simulink model "VLC_MULT"  (R2020a)
settings: Solver=VariableStepAuto  StartTime=0.0  StopTime=400  RelTol=1e-3
model workspace (MAT data in the model file):
  Name = 1
settings Model: Creator=JohnCarlo.Laude001  LastModifiedBy=JohnCarlo.Laude001

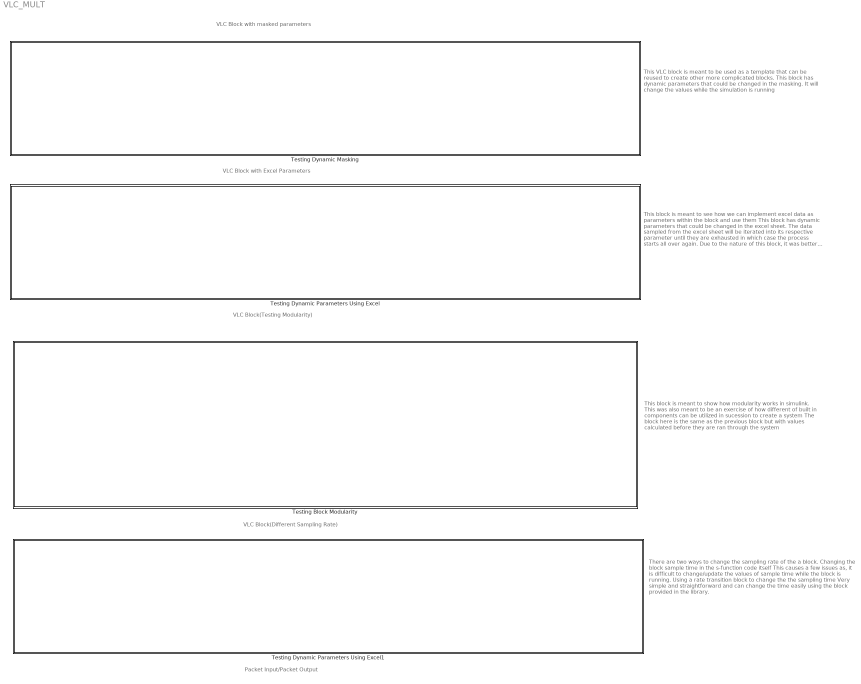
== system VLC_MULT ==
  note: This VLC block is meant to be used as a template that can be
      | reused to create other more complicated blocks.
      |
      | This block has dynamic parameters that could be changed in
      | the masking. It will change the values while the simulation is
      | running
  note: VLC Block with masked parameters
  note: VLC Block with Excel Parameters
  note: VLC Block(Testing Modularity)
  note: This block is meant to see how we can implement excel
      | data as parameters within the block and use them
      |
      | This block has dynamic parameters that could be changed in
      | the excel sheet. The data sampled from the excel sheet will be
      | iterated into its respective parameter until they are exhausted
      | in which case the process starts all over again. Due to the
      | nature of this block, it was better to run run the parameters
      | straight as inputs for ease of access instead of parameters.
  note: This block is meant to show how modularity works in simulink.
      | This was also meant to be an exercise of how different
      | of built in components can be utilized in sucession to
      | create a system
      |
      | The block here is the same as the previous block but with
      | values calculated before they are ran through the system
  note: VLC Block(Different Sampling Rate)
  note: There are two ways to change the sampling rate of the a block.
      | Changing the block sample time in the s-function code itself
      | This causes a few issues as, it is difficult to change/update
      | the values of sample time while the block is running.
      | Using a rate transition block to change the the sampling time
      | Very simple and straightforward and can change the time
      | easily using the block provided in the library.
  note: Packet Input/Packet Output
  Testing Block Modularity : Subsystem
  Testing Dynamic Masking : Subsystem
  Testing Dynamic Parameters Using Excel : Subsystem
  Testing Dynamic Parameters Using Excel1 : Subsystem

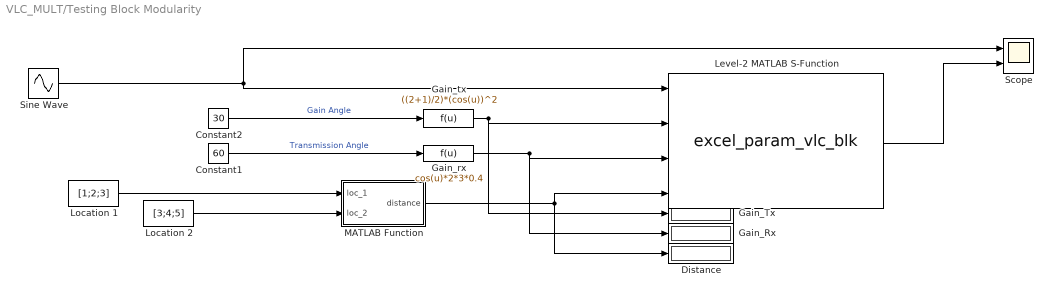
== system VLC_MULT/Testing Block Modularity ==
  Constant1 : Constant  Value=60
  Constant2 : Constant  Value=30
  Distance : Display
  Gain_Rx : Display
  Gain_Tx : Display
  Gain_rx : Fcn  Expr=cos(u)*2*3*0.4
  Gain_tx : Fcn  Expr=((2+1)/2)*(cos(u))^2
  Level-2 MATLAB S-Function : M-S-Function  FunctionName=excel_param_vlc_blk  Parameters=grx, gtx, d  mask{grx=90.0, gtx=100.0, d=100.0}
      mask prompts: grx "Gain Received"; gtx "Gain Transmission"; d "Distance"
      mask DialogControl DescGroupVar Prompt: VLC Block
      mask DialogControl DescTextVar Prompt: This block is meant to simulate the VLC system using the equation        H = (gain_tx*gain_rx)/(distance^2)
  Location 1 : Constant  Value=[1;2;3]
  Location 2 : Constant  Value=[3;4;5]
  MATLAB Function : MATLAB Function  TreatAsAtomicUnit=on
  Scope : Scope  NumInputPorts=2
  Sine Wave : Sin  SampleTime=0.001
  wires:
  Level-2 MATLAB S-Function/1 -> Scope/2
  Sine Wave/1 -> Scope/1, Level-2 MATLAB S-Function/1
  Gain_tx/1 -> Gain_Tx/1, Level-2 MATLAB S-Function/2
  Constant2/1 -> Gain_tx/1  "Gain Angle"
  Constant1/1 -> Gain_rx/1  "Transmission Angle"
  Gain_rx/1 -> Level-2 MATLAB S-Function/3, Gain_Rx/1
  Location 1/1 -> MATLAB Function/1(loc_1)
  MATLAB Function/1(distance) -> Level-2 MATLAB S-Function/4, Distance/1
  Location 2/1 -> MATLAB Function/2(loc_2)

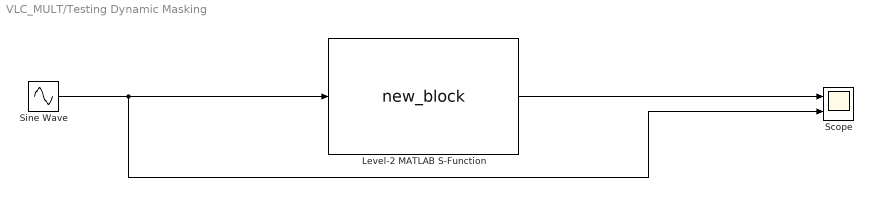
== system VLC_MULT/Testing Dynamic Masking ==
  Level-2 MATLAB S-Function : M-S-Function  FunctionName=new_block  Parameters=grx, gtx, d  mask{grx=81.0, gtx=41.0, d=78.0}
      mask prompts: grx "Gain Received"; gtx "Gain Transmission"; d "Distance"
      mask DialogControl DescGroupVar Prompt: VLC Block
      mask DialogControl DescTextVar Prompt: This block is meant to simulate the VLC system using the equation        H = (gain_tx*gain_rx)/(distance^2)
  Scope : Scope  NumInputPorts=2
  Sine Wave : Sin  SampleTime=0.001
  wires:
  Level-2 MATLAB S-Function/1 -> Scope/1
  Sine Wave/1 -> Scope/2, Level-2 MATLAB S-Function/1

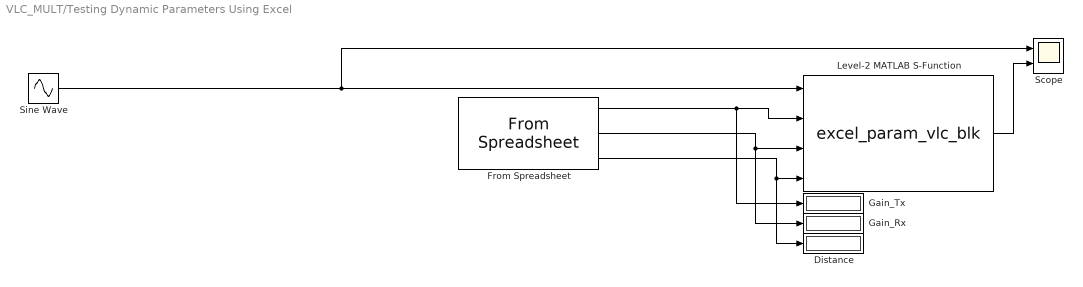
== system VLC_MULT/Testing Dynamic Parameters Using Excel ==
  Distance : Display
  From Spreadsheet : FromSpreadsheet  FileName=C:\Users\JohnCarlo.Laude001\Desktop\VLC_Research\VLC_Data_Test.xlsx  TreatFirstColumnAs=Data  SampleTime=50
  Gain_Rx : Display
  Gain_Tx : Display
  Level-2 MATLAB S-Function : M-S-Function  FunctionName=excel_param_vlc_blk  Parameters=grx, gtx, d  mask{grx=18.900, gtx=100.0, d=100.0}
      mask prompts: grx "Gain Received"; gtx "Gain Transmission"; d "Distance"
      mask DialogControl DescGroupVar Prompt: VLC Block
      mask DialogControl DescTextVar Prompt: This block is meant to simulate the VLC system using the equation        H = (gain_tx*gain_rx)/(distance^2)
  Scope : Scope  NumInputPorts=2
  Sine Wave : Sin  SampleTime=0.001
  wires:
  Sine Wave/1 -> Scope/1, Level-2 MATLAB S-Function/1
  From Spreadsheet/1 -> Gain_Tx/1, Level-2 MATLAB S-Function/2
  From Spreadsheet/2 -> Gain_Rx/1, Level-2 MATLAB S-Function/3
  From Spreadsheet/3 -> Distance/1, Level-2 MATLAB S-Function/4
  Level-2 MATLAB S-Function/1 -> Scope/2

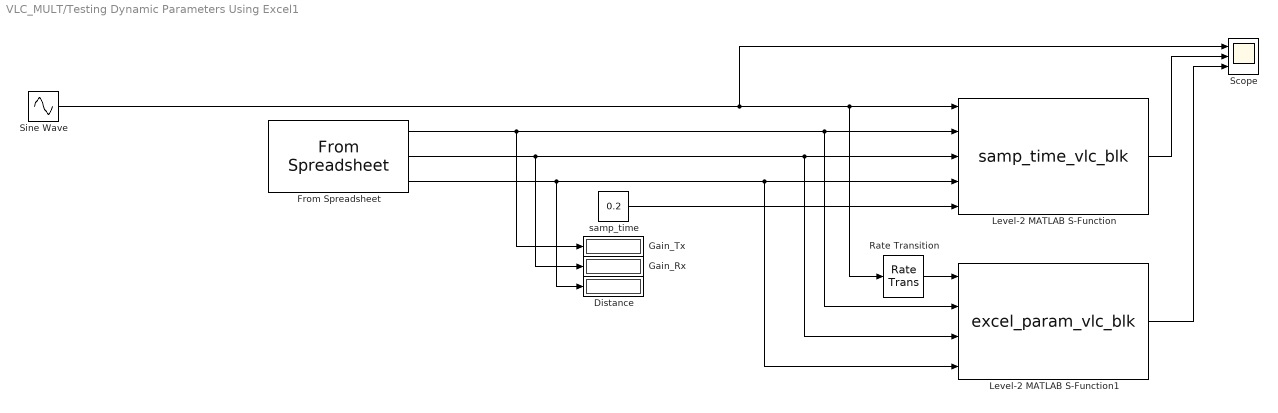
== system VLC_MULT/Testing Dynamic Parameters Using Excel1 ==
  Distance : Display
  From Spreadsheet : FromSpreadsheet  FileName=C:\Users\JohnCarlo.Laude001\Desktop\VLC_Research\VLC_Data_Test.xlsx  TreatFirstColumnAs=Data  SampleTime=1000
  Gain_Rx : Display
  Gain_Tx : Display
  Level-2 MATLAB S-Function : M-S-Function  FunctionName=samp_time_vlc_blk  Parameters=grx, gtx, d  mask{grx=18.900, gtx=100.0, d=100.0}
      mask prompts: grx "Gain Received"; gtx "Gain Transmission"; d "Distance"
      mask DialogControl DescGroupVar Prompt: VLC Block
      mask DialogControl DescTextVar Prompt: This block is meant to simulate the VLC system using the equation        H = (gain_tx*gain_rx)/(distance^2)
  Level-2 MATLAB S-Function1 : M-S-Function  FunctionName=excel_param_vlc_blk  Parameters=grx, gtx, d  mask{grx=18.900, gtx=100.0, d=100.0}
      mask prompts: grx "Gain Received"; gtx "Gain Transmission"; d "Distance"
      mask DialogControl DescGroupVar Prompt: VLC Block
      mask DialogControl DescTextVar Prompt: This block is meant to simulate the VLC system using the equation        H = (gain_tx*gain_rx)/(distance^2)
  Rate Transition : RateTransition  OutPortSampleTime=0.5
  Scope : Scope  NumInputPorts=3
  Sine Wave : Sin  SampleTime=0.001
  samp_time : Constant  Value=0.2
  wires:
  From Spreadsheet/1 -> Gain_Tx/1, Level-2 MATLAB S-Function1/2, Level-2 MATLAB S-Function/2
  From Spreadsheet/2 -> Gain_Rx/1, Level-2 MATLAB S-Function1/3, Level-2 MATLAB S-Function/3
  From Spreadsheet/3 -> Distance/1, Level-2 MATLAB S-Function1/4, Level-2 MATLAB S-Function/4
  Sine Wave/1 -> Scope/1, Rate Transition/1, Level-2 MATLAB S-Function/1
  Level-2 MATLAB S-Function/1 -> Scope/2
  samp_time/1 -> Level-2 MATLAB S-Function/5
  Rate Transition/1 -> Level-2 MATLAB S-Function1/1
  Level-2 MATLAB S-Function1/1 -> Scope/3

== matlab function VLC_MULT/Testing Block Modularity/MATLAB Function ==
  data: loc_1 input; distance output; loc_2 input
function distance = fcn(loc_1,loc_2)
% Calculate the distance of two 3D points using the equation for
% Euclidian distance.
distance = sqrt(sum((loc_1 - loc_2).^2))
